simulink model "whole_circuit"  (R2023b)
settings: Solver=VariableStepAuto  StartTime=0.0  StopTime=0.2  RelTol=1e-3
libraries: spsDiodeLib x7, spsVoltageMeasurementLib x6, spsCurrentMeasurementLib x5, spsSeriesRLCBranchLib x4, spsMosfetLib x1, spsThreePhaseSourceLib x1, sps_lib x1
settings Model: Creator=gencb  LastModifiedBy=gencb

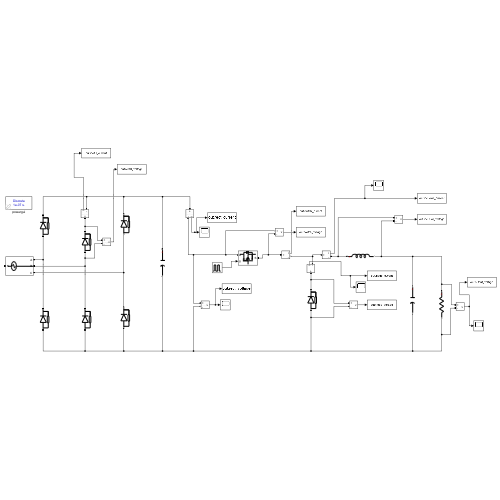
[thumbnail: Simulink's stored preview of the top-level diagram]
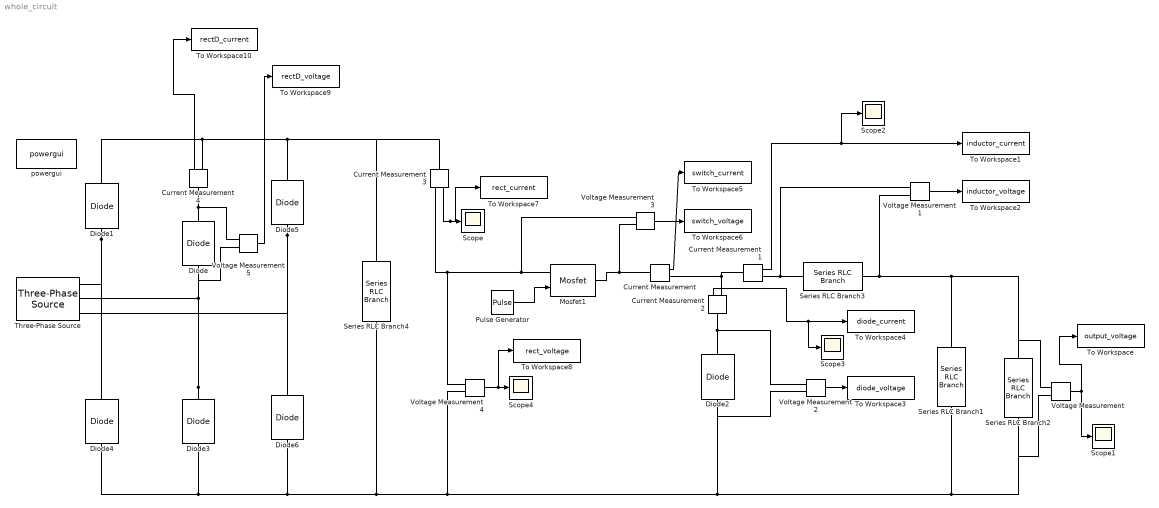
== system whole_circuit ==
  Current Measurement{,1..4} (5 alike) : spsCurrentMeasurementLib/Current Measurement  PhasorSimulation=off  OutputType=Complex  PSBequivalent=0
  Diode{,1,3..6} (6 alike) : spsDiodeLib/Diode  Ron=0.001  Lon=0  Vf=0.1  IC=0  UseSnubber=0  Rs=500  Cs=250e-9  Measurements=off
  Diode2 : spsDiodeLib/Diode  Ron=0.001  Lon=0  Vf=0.01  IC=0  UseSnubber=0  Rs=500  Cs=250e-9  Measurements=off
  Mosfet1 : spsMosfetLib/Mosfet  Ron=0.01  Lon=0  Rd=0.001  Vfd=0  IC=0  Rs=1e5  Cs=inf  Measurements=off
  Pulse Generator : DiscretePulseGenerator  PulseType=Time based  Period=1/80000  PulseWidth=34
  Scope{,1..4} (5 alike) : Scope
  Series RLC Branch1 : spsSeriesRLCBranchLib/Series RLC Branch  LConnTagsString=__new0  RConnTagsString=__new0  BranchType=C  Resistance=1  Inductance=76.8e-6  SetiL0=off  InitialCurrent=0  Capacitance=13e-6  Setx0=off  InitialVoltage=0  Measurements=None
  Series RLC Branch2 : spsSeriesRLCBranchLib/Series RLC Branch  LConnTagsString=__new0  RConnTagsString=__new0  BranchType=R  Resistance=1.2  Inductance=76.8e-6  SetiL0=off  InitialCurrent=0  Capacitance=400e-6  Setx0=off  InitialVoltage=0  Measurements=None
  Series RLC Branch3 : spsSeriesRLCBranchLib/Series RLC Branch  LConnTagsString=__new0  RConnTagsString=__new0  BranchType=L  Resistance=1  Inductance=65e-6  SetiL0=off  InitialCurrent=0  Capacitance=1e-6  Setx0=off  InitialVoltage=0  Measurements=None
  Series RLC Branch4 : spsSeriesRLCBranchLib/Series RLC Branch  LConnTagsString=__new0  RConnTagsString=__new0  BranchType=C  Resistance=1  Inductance=1e-3  SetiL0=off  InitialCurrent=0  Capacitance=2200e-6  Setx0=off  InitialVoltage=0  Measurements=None
  Three-Phase Source : spsThreePhaseSourceLib/Three-Phase Source  InternalConnection=Yn  VoltagePhases=off  Voltage=25  PhaseAngle=0  Voltage_phases=[25e3 25e3 25e3]/sqrt(3)  PhaseAngles_phases=[0 -120 +120]  Frequency=50  NonIdealSource=on  SpecifyImpedance=off  Resistance=0  Inductance=0  ShortCircuitLevel=100e6  BaseVoltage=25  XRratio=7  BusType=swing  Pref=10e3  Qref=0  Prefabc=[10e3, 10e3, 10e3]  Qrefabc=[0, 0, 0]  Qmin=-inf  Qmax=inf
  To Workspace : ToWorkspace  VariableName=output_voltage  SaveFormat=Timeseries  SampleTime=-1
  To Workspace1 : ToWorkspace  VariableName=inductor_current  SaveFormat=Timeseries  SampleTime=-1
  To Workspace10 : ToWorkspace  VariableName=rectD_current  SaveFormat=Timeseries  SampleTime=-1
  To Workspace2 : ToWorkspace  VariableName=inductor_voltage  SaveFormat=Timeseries  SampleTime=-1
  To Workspace3 : ToWorkspace  VariableName=diode_voltage  SaveFormat=Timeseries  SampleTime=-1
  To Workspace4 : ToWorkspace  VariableName=diode_current  SaveFormat=Timeseries  SampleTime=-1
  To Workspace5 : ToWorkspace  VariableName=switch_current  SaveFormat=Timeseries  SampleTime=-1
  To Workspace6 : ToWorkspace  VariableName=switch_voltage  SaveFormat=Timeseries  SampleTime=-1
  To Workspace7 : ToWorkspace  VariableName=rect_current  SaveFormat=Timeseries  SampleTime=-1
  To Workspace8 : ToWorkspace  VariableName=rect_voltage  SaveFormat=Timeseries  SampleTime=-1
  To Workspace9 : ToWorkspace  VariableName=rectD_voltage  SaveFormat=Timeseries  SampleTime=-1
  Voltage Measurement{,1..5} (6 alike) : spsVoltageMeasurementLib/Voltage Measurement  PhasorSimulation=off  OutputType=Complex  PSBequivalent=0
  powergui : sps_lib/powergui  Priority=1  SimulationMode=Discrete  SampleTime=0.1e-6  frequency=60  Iterations=50  frequencyindice=0  Pbase=100e6  ErrMax=1e-4  UnitsV=kV  UnitsW=MW  buscounter=0  FunctionMessages=off  echomessages=off  EnableUseOfTLC=off  CurrentSourceSwitches=off  DisableSnubberDevices=off  DisableRonSwitches=off  DisableVfSwitches=off  DisplayEquations=off  AutomaticDiscreteSolvers=off  SolverType=Tustin/Backward Euler (TBE)  Interpol=off  ExternalGateDelay=off  methode=off  Ts=100  x0status=blocks  SPID=on  SwTol=0  HookPort=off  NonlinearTolerance=1e-4  nMaxIteration=100  ContinueOnMaxIteration=off  RestoreLinks=warning  ResistiveCurrentMeasurement=off  Frange=[0:2:500]  Ylog=off  Xlog=on  ShowGrid=off  save=off  variable=ZData  structure=0  ZoomFFT=off  StartTime=0.0  cycles=1  DisplayStyle=1  fundamental=60  FreqAxis=off  MaxFrequency=1000  frequencyindicesteady=1  RmsSteady=1  display=off
  wires:
  Voltage Measurement2/1 -> To Workspace3/1
  Current Measurement1/1 -> Scope2/1, To Workspace1/1
  Voltage Measurement1/1 -> To Workspace2/1
  Voltage Measurement3/1 -> To Workspace6/1
  Current Measurement/1 -> To Workspace5/1
  Pulse Generator/1 -> Mosfet1/1
  Current Measurement2/1 -> Scope3/1, To Workspace4/1
  Voltage Measurement4/1 -> To Workspace8/1, Scope4/1
  Current Measurement3/1 -> To Workspace7/1, Scope/1
  Voltage Measurement/1 -> To Workspace/1, Scope1/1
  Current Measurement4/1 -> To Workspace10/1
  Voltage Measurement5/1 -> To Workspace9/1
  connections:
  Voltage Measurement3/LConn2 -- Mosfet1/RConn1 -- Current Measurement/LConn1
  Series RLC Branch4/RConn1 -- Diode2/LConn1 -- Voltage Measurement2/LConn2 -- Series RLC Branch2/RConn1 -- Voltage Measurement/LConn2 -- Series RLC Branch1/RConn1 -- Voltage Measurement4/LConn2 -- Diode6/LConn1 -- Diode3/LConn1 -- Diode4/LConn1
  Current Measurement3/RConn1 -- Voltage Measurement4/LConn1 -- Voltage Measurement3/LConn1 -- Mosfet1/LConn1
  Voltage Measurement1/LConn2 -- Series RLC Branch2/LConn1 -- Voltage Measurement/LConn1 -- Series RLC Branch1/LConn1 -- Series RLC Branch3/RConn1
  Diode2/RConn1 -- Current Measurement2/LConn1 -- Voltage Measurement2/LConn1
  Current Measurement/RConn1 -- Current Measurement1/LConn1 -- Current Measurement2/RConn1
  Current Measurement1/RConn1 -- Series RLC Branch3/LConn1 -- Voltage Measurement1/LConn1
  Diode1/LConn1 -- Three-Phase Source/RConn1 -- Diode4/RConn1
  Diode3/RConn1 -- Diode/LConn1 -- Voltage Measurement5/LConn2 -- Three-Phase Source/RConn2
  Current Measurement3/LConn1 -- Series RLC Branch4/LConn1 -- Diode5/RConn1 -- Current Measurement4/RConn1 -- Diode1/RConn1
  Diode5/LConn1 -- Diode6/RConn1 -- Three-Phase Source/RConn3
  Current Measurement4/LConn1 -- Voltage Measurement5/LConn1 -- Diode/RConn1
